simulink model "BNO055"  (R2021b)
settings: Solver=FixedStepAuto  StartTime=0.0  StopTime=Inf  FixedStep=0.02  RelTol=1e-3  EnableMultiTasking=on
settings Model: ExtModeTrigDuration=8  LastModifiedBy=NRPU
settings OptimizationCC: DefaultUnderspecifiedDataType=single  EnhancedBackFolding=on  PassReuseOutputArgsAs=Individual arguments  MaxStackSize=1024  OptimizeBlockOrder=speed  DifferentSizesBufferReuse=on  OptimizationCustomize=off  DenormalBehavior=FlushToZero  EfficientTunableParamExpr=on
settings DebuggingCC: ParameterTunabilityLossMsg=error
settings HardwareCC: ProdBitPerChar=16  ProdBitPerInt=16  ProdBitPerPointer=32  ProdBitPerSizeT=32  ProdBitPerPtrDiffT=32  ProdLargestAtomicInteger=Integer  ProdLargestAtomicFloat=None  ProdWordSize=16  ProdLongLongMode=on  ProdHWDeviceType=Texas Instruments->C2000
settings ModelReferenceCC: ModelReferenceNumInstancesAllowed=Single
settings SFSimCC: MATLABDynamicMemAlloc=off
settings RTWCC: Description=Embedded Coder  SystemTargetFile=ert.tlc  HardwareBoard=TI Delfino F28379D LaunchPad  TemplateMakefile=ert_default_tmf  Toolchain=Texas Instruments Code Composer Studio (C2000)
settings CodeAppCC: ForceParamTrailComments=on  IgnoreCustomStorageClasses=off  OperatorAnnotations=on  SimulinkDataObjDesc=on  SFDataObjDesc=on  InsertBlockDesc=on
settings ERTTargetCC: CodeReplacementLibrary=TI C28x  SupportContinuousTime=on  ExtModeTransport=4  ExtModeStaticAlloc=on  ExtModeStaticAllocSize=10000  ExtModeMexFile=ext_xcp  ExtModeIntrfLevel=Level2 - Open

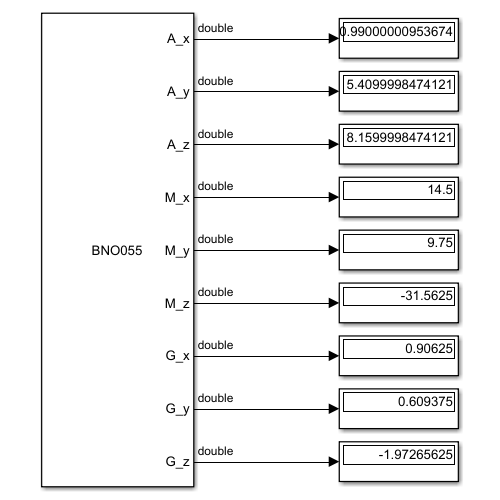
[thumbnail: Simulink's stored preview of the top-level diagram]
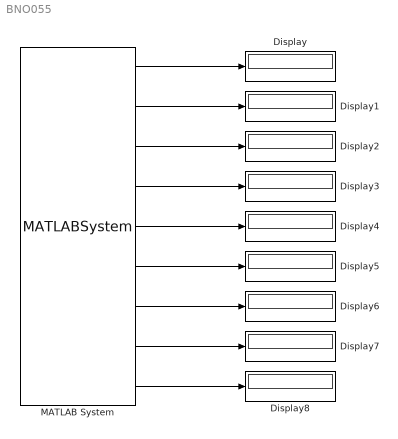
== system BNO055 ==
  Display{,1..8} (9 alike) : Display
  MATLAB System : MATLABSystem  System=BNO055_block
      mask Type: BNO055_block
      mask Display:
      | disp('BNO055');
      | port_label('output',1,'A_x');
      | port_label('output',2,'A_y');
      | port_label('output',3,'A_z');
      | port_label('output',4,'M_x');
      | port_label('output',5,'M_y');
      | port_label('output',6,'M_z');
      | port_label('output',7,'G_x');
      | port_label('output',8,'G_y');
      | port_label('output',9,'G_z');
  wires:
  MATLAB System/6 -> Display5/1
  MATLAB System/2 -> Display1/1
  MATLAB System/1 -> Display/1
  MATLAB System/5 -> Display4/1
  MATLAB System/4 -> Display3/1
  MATLAB System/3 -> Display2/1
  MATLAB System/7 -> Display6/1
  MATLAB System/8 -> Display7/1
  MATLAB System/9 -> Display8/1
